simulink model "model1"  (R2020b)
settings: Solver=ode1  StartTime=0.0  StopTime=20.0  FixedStep=dt  RelTol=1e-3
values from neighbouring files (symbols this model uses):
  b = 45    [haptic_interface.m]
  K = 1    [haptic_interface.m]
  k = 1    [haptic_interface.m]
  m = 15    [haptic_interface.m]
  object_b = 2.5    [haptic_interface.m]
  object_k = 5    [haptic_interface.m]
  object_width = 20    [haptic_interface.m]
settings Model: Creator=berke  LastModifiedBy=berke

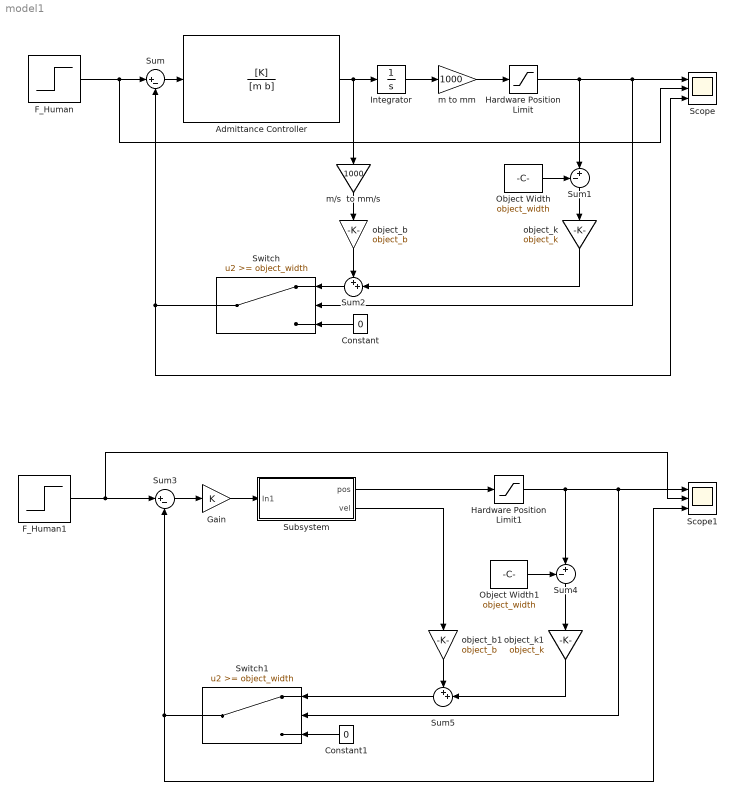
== system model1 ==
  Admittance Controller : TransferFcn  Numerator=[K]  Denominator=[m b]
  Constant : Constant  Value=0
  Constant1 : Constant  Value=0
  F_Human : Step  SampleTime=0
  F_Human1 : Step  SampleTime=0
  Gain : Gain  Gain=K
  Hardware Position Limit : Saturate  UpperLimit=40  LowerLimit=0
  Hardware Position Limit1 : Saturate  UpperLimit=40  LowerLimit=0
  Integrator : Integrator
  Object Width : Constant  Value=object_width
  Object Width1 : Constant  Value=object_width
  Scope : Scope  NumInputPorts=3
  Scope1 : Scope  NumInputPorts=3
  Subsystem : Subsystem
  Sum : Sum  Inputs=|+-
  Sum1 : Sum  Inputs=-+|
  Sum2 : Sum  Inputs=++|
  Sum3 : Sum  Inputs=|+-
  Sum4 : Sum  Inputs=-+|
  Sum5 : Sum  Inputs=++|
  Switch : Switch  Threshold=object_width
  Switch1 : Switch  Threshold=object_width
  m to mm : Gain  Gain=1000
  m/s  to mm/s : Gain  Gain=1000
  object_b : Gain  Gain=object_b
  object_b1 : Gain  Gain=object_b
  object_k : Gain  Gain=object_k
  object_k1 : Gain  Gain=object_k
  wires:
  Sum/1 -> Admittance Controller/1
  F_Human/1 -> Scope/2, Sum/1
  Admittance Controller/1 -> m/s  to mm/s/1, Integrator/1
  Integrator/1 -> m to mm/1
  m to mm/1 -> Hardware Position Limit/1
  Hardware Position Limit/1 -> Scope/1, Switch/2, Sum1/2
  Switch/1 -> Scope/3, Sum/2
  Constant/1 -> Switch/3
  m/s  to mm/s/1 -> object_b/1
  Sum1/1 -> object_k/1
  Object Width/1 -> Sum1/1
  object_b/1 -> Sum2/1
  Sum2/1 -> Switch/1
  object_k/1 -> Sum2/2
  object_b1/1 -> Sum5/1
  Sum5/1 -> Switch1/1
  Object Width1/1 -> Sum4/1
  Constant1/1 -> Switch1/3
  Sum4/1 -> object_k1/1
  Subsystem/2(vel) -> object_b1/1
  Switch1/1 -> Sum3/2, Scope1/3
  Subsystem/1(pos) -> Hardware Position Limit1/1
  object_k1/1 -> Sum5/2
  F_Human1/1 -> Scope1/2, Sum3/1
  Hardware Position Limit1/1 -> Scope1/1, Switch1/2, Sum4/2
  Gain/1 -> Subsystem/1(In1)
  Sum3/1 -> Gain/1

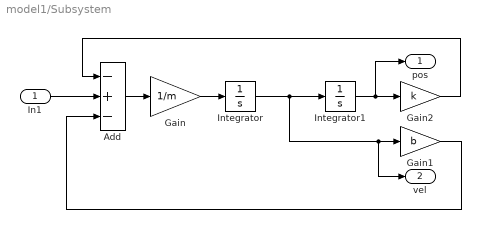
== system model1/Subsystem ==
  In1 : Inport
  Add : Sum  Inputs=-+-
  Gain : Gain  Gain=1/m
  Gain1 : Gain  Gain=b
  Gain2 : Gain  Gain=k
  Integrator : Integrator
  Integrator1 : Integrator
  pos : Outport
  vel : Outport  Port=2
  wires:
  Integrator/1 -> Integrator1/1, vel/1, Gain1/1
  Gain1/1 -> Add/3
  Integrator1/1 -> pos/1, Gain2/1
  Gain2/1 -> Add/1
  Add/1 -> Gain/1
  Gain/1 -> Integrator/1
  In1/1 -> Add/2
